simulink subsystem "Controller_Subsystem"  (R2022b)
settings: Solver=VariableStepAuto  StartTime=0.0  StopTime=10.0  RelTol=1e-3
settings Model: Creator=Sahil Gaurkar  LastModifiedBy=Sahil Gaurkar

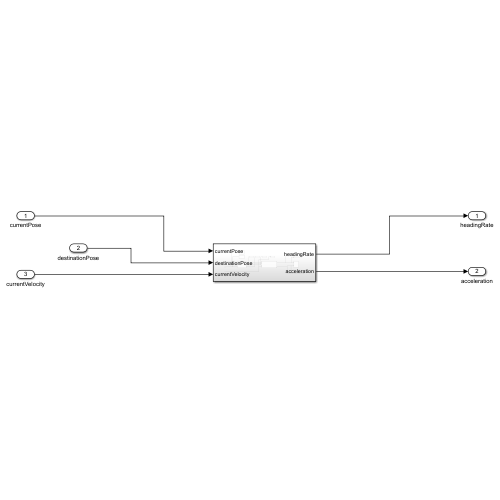
[thumbnail: Simulink's stored preview of the top-level diagram]
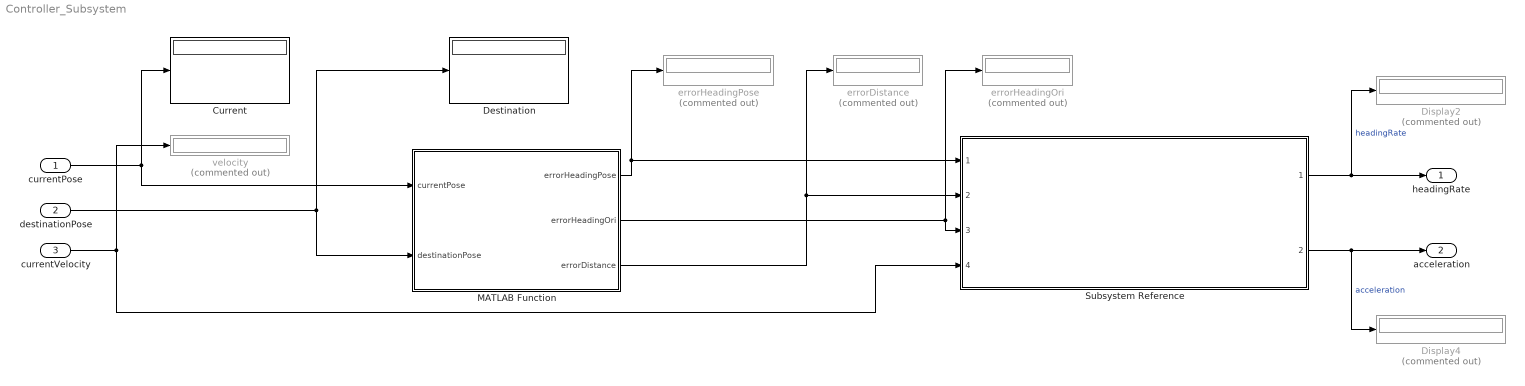
== system Controller_Subsystem ==
  currentPose : Inport
  destinationPose : Inport  Port=2
  currentVelocity : Inport  Port=3
  Current : Display
  Destination : Display
  Display2 : Display  Commented=on
  Display4 : Display  Commented=on
  MATLAB Function : MATLAB Function  TreatAsAtomicUnit=on
  Subsystem Reference : Subsystem  ReferencedSubsystem=Controller
  errorDistance : Display  Commented=on
  errorHeadingOri : Display  Commented=on
  errorHeadingPose : Display  Commented=on
  velocity : Display  Commented=on
  headingRate : Outport
  acceleration : Outport  Port=2
  wires:
  currentPose/1 -> MATLAB Function/1(currentPose), Current/1
  Subsystem Reference/2 -> acceleration/1, Display4/1  "acceleration"
  MATLAB Function/3(errorDistance) -> errorDistance/1, Subsystem Reference/2
  MATLAB Function/1(errorHeadingPose) -> errorHeadingPose/1, Subsystem Reference/1
  MATLAB Function/2(errorHeadingOri) -> Subsystem Reference/3, errorHeadingOri/1
  Subsystem Reference/1 -> headingRate/1, Display2/1  "headingRate"
  currentVelocity/1 -> Subsystem Reference/4, velocity/1
  destinationPose/1 -> MATLAB Function/2(destinationPose), Destination/1

== matlab function Controller_Subsystem/MATLAB Function ==
  data: currentPose input; errorHeadingPose output; errorHeadingOri output; destinationPose input; errorDistance output
function [errorHeadingPose, errorHeadingOri, errorDistance] = fcn(currentPose, destinationPose)

errorDistance = 0;
errorHeadingPose = 0;
errorHeadingOri = 0;


errorDistance = sqrt( (destinationPose(1)-currentPose(1))^2 + (destinationPose(2)-currentPose(2))^2 );
errorHeadingPose = atan2d(destinationPose(2) - currentPose(2), destinationPose(1) - currentPose(1)) - currentPose(3);


if abs(errorHeadingPose) > 1 && abs(errorDistance) > 1
    errorHeadingPose = atan2d(destinationPose(2) - currentPose(2), destinationPose(1) - currentPose(1)) - currentPose(3);
    errorHeadingOri = 0;
    errorDistance = 0;
elseif abs(errorDistance) > 1
    errorDistance = sqrt( (destinationPose(1)-currentPose(1))^2 + (destinationPose(2)-currentPose(2))^2 );
    errorHeadingOri = 0; 
   errorHeadingPose = atan2d(destinationPose(2) - currentPose(2), destinationPose(1) - currentPose(1)) - currentPose(3);
else
    errorHeadingOri = destinationPose(3) - currentPose(3);
    errorHeadingPose = 0;
    errorDistance = 0;
end



end
